simulink model "simulation_scalar"  (R2021b)
settings: Solver=VariableStepAuto  StartTime=0.0  StopTime=6  MaxStep=0.001  RelTol=1e-3
values from neighbouring files (symbols this model uses):
  k43 = 0    [exception.mat]    (also in robustness.mat = 663.324958071; scalar.mat = 61.6408497202; scalar_net.m = sqrt(2)*omega43*sqrt(abs(M(4,3)/M(3,4))); scalar_net_CreationNewConnection.m = sqrt(2)*omega43*sqrt(abs(M(4,3)/M(3,4))))
  k43_2 = 54.3557306505    [scalar.mat]
  k51 = 946.044396421    [exception.mat]    (also in robustness.mat = 146.385010942; scalar.mat = 259.670461528; scalar_net.m = sqrt(2)*omega51*sqrt(abs(M(5,1)/M(1,5))); scalar_net_CreationNewConnection.m = sqrt(2)*omega51*sqrt(abs(M(5,1)/M(1,5))))
  k51_2 = 242.383992871    [scalar.mat]
  M = [-1.5 0 -0.7 0 17.9 0 -4.1 -6.8 0 0 0 0 ... (25 elements, 5x5)]    [exception.mat]    (also in nonscalar.mat = [-3.8 1.9 -4.5 0 0 0 -4.6 1.6 0 0 0 0 ... (25 elements, 5x5); nonscalar_net.m = round(M,1); nonscalar_net_general.m = sym('M',sum(n)); robustness.mat = [-8.5 0 -1.6 0 1.5 0 -5.3 -4.7 0 0 0 0 ... (25 elements, 5x5)
  M_bar = [-8.5 0 -1.6 0 2.22044604925e-16 0 -5.3 -4.7 0 0 0 0 ... (25 elements, 5x5)]    [robustness.mat]    (also in scalar.mat = [-1.7 0 -6.4 0 0.05 0 -4.8 -9.5 0 0 0 0 ... (25 elements, 5x; test_meerkov_nonscalar_different.m = M + B_bar; test_meerkov_nonscalar_equal.m = M + V_bar)
  M_stable = [-1.7 0 -0.64 0 0.26 0 -4.8 -0.95 0 0 0 0 ... (25 elements, 5x5)]    [scalar.mat]    (also in scalar_net.m = A+Lambda2)
  N = 5    [exception.mat]    (also in nonscalar_net.m = 3; nonscalar_net_general.m = 4; robustness.mat; scalar.mat)
  omega43 = 50    [exception.mat]    (also in robustness.mat; scalar.mat; scalar_net.m = 200; scalar_net_CreationNewConnection.m)
  omega43_2 = 50    [scalar.mat]
  omega51 = 50    [exception.mat]    (also in robustness.mat = 70.7106781187; scalar.mat = 70.7106781187; scalar_net.m = sqrt(2) * omega_0; scalar_net_CreationNewConnection.m = sqrt(2) * omega_0)
  omega51_2 = 70.7106781187    [scalar.mat]
  x_0 = [1 1 1 1 1]    [exception.mat]    (also in nonscalar_net.m = ones(sum(n),1); robustness.mat; scalar.mat; scalar_net.m = ones(5,1))
  y_0 = double(inv_F0*x_0)    [nonscalar_net.m]    (also in scalar_net.m)
settings Model: Creator=alber  LastModifiedBy=anobili

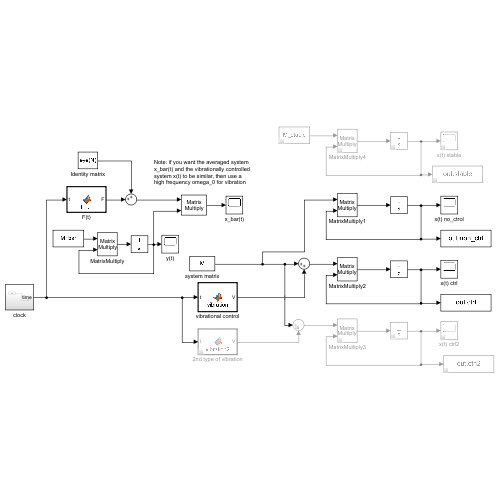
[thumbnail: Simulink's stored preview of the top-level diagram]
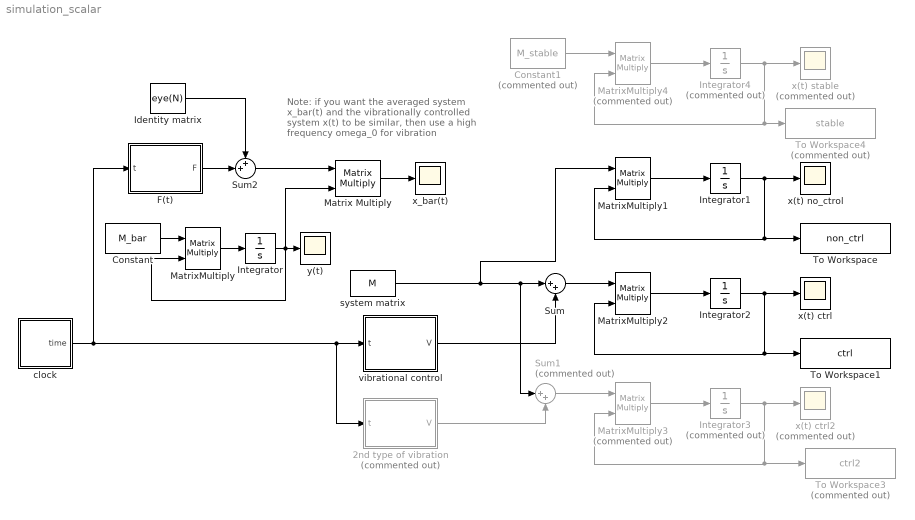
== system simulation_scalar ==
  note: Note: if you want the averaged system x_bar(t) and the vibrationally controlled system x(t) to be similar, then use a high frequency omega_0 for vibration
  2nd type of vibration : MATLAB Function  Commented=on  TreatAsAtomicUnit=on
  Constant : Constant  Value=M_bar
  Constant1 : Constant  Commented=on  Value=M_stable
  F(t) : MATLAB Function  TreatAsAtomicUnit=on
  Identity matrix : Constant  Value=eye(N)
  Integrator : Integrator  InitialCondition=y_0
  Integrator1 : Integrator  InitialCondition=x_0
  Integrator2 : Integrator  InitialCondition=x_0
  Integrator3 : Integrator  Commented=on  InitialCondition=x_0
  Integrator4 : Integrator  Commented=on  InitialCondition=x_0
  Matrix Multiply : Product  Multiplication=Matrix(*)
  MatrixMultiply : Product  Multiplication=Matrix(*)
  MatrixMultiply1 : Product  Multiplication=Matrix(*)
  MatrixMultiply2 : Product  Multiplication=Matrix(*)
  MatrixMultiply3 : Product  Commented=on  Multiplication=Matrix(*)
  MatrixMultiply4 : Product  Commented=on  Multiplication=Matrix(*)
  Sum : Sum  Inputs=|++
  Sum1 : Sum  Commented=on  Inputs=|++
  Sum2 : Sum  Inputs=++|
  To Workspace : ToWorkspace  VariableName=non_ctrl  SaveFormat=Timeseries  SampleTime=-1
  To Workspace1 : ToWorkspace  VariableName=ctrl  SaveFormat=Timeseries  SampleTime=-1
  To Workspace3 : ToWorkspace  Commented=on  VariableName=ctrl2  SaveFormat=Timeseries  SampleTime=-1
  To Workspace4 : ToWorkspace  Commented=on  VariableName=stable  SaveFormat=Timeseries  SampleTime=-1
  clock : Subsystem
  system matrix : Constant  Value=M
  vibrational control : MATLAB Function  TreatAsAtomicUnit=on
  x(t) ctrl : Scope
  x(t) ctrl2 : Scope  Commented=on
  x(t) no_ctrol : Scope
  x(t) stable : Scope  Commented=on
  x_bar(t) : Scope
  y(t) : Scope
  wires:
  Constant/1 -> MatrixMultiply/1
  Integrator/1 -> Matrix Multiply/2, y(t)/1, MatrixMultiply/2
  MatrixMultiply/1 -> Integrator/1
  MatrixMultiply1/1 -> Integrator1/1
  Integrator1/1 -> x(t) no_ctrol/1, MatrixMultiply1/2, To Workspace/1
  Integrator2/1 -> x(t) ctrl/1, To Workspace1/1, MatrixMultiply2/2
  MatrixMultiply2/1 -> Integrator2/1
  Sum/1 -> MatrixMultiply2/1
  vibrational control/1(V) -> Sum/2
  2nd type of vibration/1(V) -> Sum1/2
  Integrator3/1 -> x(t) ctrl2/1, To Workspace3/1, MatrixMultiply3/2
  clock/1(time) -> F(t)/1(t), 2nd type of vibration/1(t), vibrational control/1(t)
  MatrixMultiply3/1 -> Integrator3/1
  Sum1/1 -> MatrixMultiply3/1
  system matrix/1 -> Sum1/1, Sum/1, MatrixMultiply1/1
  Integrator4/1 -> x(t) stable/1, MatrixMultiply4/2, To Workspace4/1
  Constant1/1 -> MatrixMultiply4/1
  MatrixMultiply4/1 -> Integrator4/1
  Sum2/1 -> Matrix Multiply/1
  F(t)/1(F) -> Sum2/2
  Identity matrix/1 -> Sum2/1
  Matrix Multiply/1 -> x_bar(t)/1

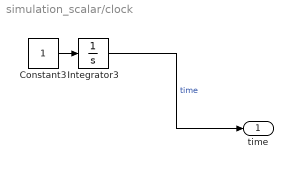
== system simulation_scalar/clock ==
  Constant3 : Constant
  Integrator3 : Integrator
  time : Outport
  wires:
  Constant3/1 -> Integrator3/1
  Integrator3/1 -> time/1  "time"

== matlab function simulation_scalar/2nd type of vibration ==
  data: t input; V output; omega43_2 parameter; k43_2 parameter; omega51_2 parameter; k51_2 parameter
function V = vibration2(t, omega43_2, k43_2, omega51_2, k51_2)

V = zeros(5);
V(5,1) = k51_2*sin(omega51_2*t);
V(4,3) = k43_2*sin(omega43_2*t);

== matlab function simulation_scalar/vibrational control ==
  data: t input; V output; omega43 parameter; k43 parameter; omega51 parameter; k51 parameter
function V = vibration(t, omega43, k43, omega51, k51)

V = zeros(5);
V(5,1) = k51*sin(omega51*t);
V(4,3) = k43*sin(omega43*t);

== matlab function simulation_scalar/F(t) ==
  data: t input; F output
function F = F_t_(t)
%#codegen

%    This function was generated by the Symbolic Math Toolbox version 9.0.
%    26-Sep-2022 10:39:48

F = reshape([0.0,0.0,0.0,0.0,sqrt(2.1e+1).*sqrt(6.7e+1).*cos(t.*7.071067811865476e+2).*(-2.0./6.7e+1),0.0,0.0,0.0,0.0,0.0,0.0,0.0,0.0,sqrt(2.3e+1).*sqrt(4.3e+1).*cos(t.*5.0e+2).*(-1.0./4.3e+1),0.0,0.0,0.0,0.0,0.0,0.0,0.0,0.0,0.0,0.0,0.0],[5,5]);
